simulink model "simulation"  (R2017b)
settings: Solver=FixedStepAuto  StartTime=0.0  StopTime=simTotalTime  FixedStep=0.05  MaxStep=0.1  MinStep=0.01  RelTol=1e-3
undefined symbols (not defined in the file): gridArea, gridDen, gridLength, hysteronMax, hysteronMin, initialRelays, inputFactor, inputMax, inputMin, offset, outputFactor, outputMax, outputMin, weightFunc, xyGrid
libraries: simulink x1
settings Model: Creator=Marco  LastModifiedBy=M. Vasquez Beltran

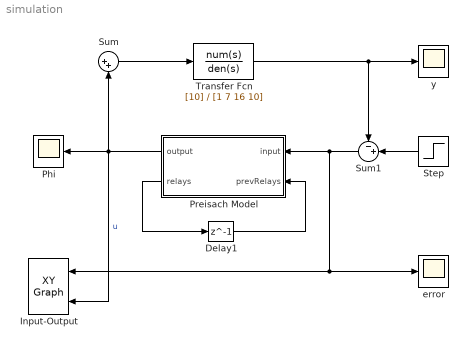
== system simulation ==
  Delay1 : Delay  DelayLength=1  InitialCondition=initialRelays
  Input-Output : simulink/Sinks/XY Graph  xmin=inputMin*inputFactor  xmax=inputMax*inputFactor  ymin=outputMin*outputFactor  ymax=outputMax*outputFactor  st=-1
  Phi : Scope
  Preisach Model : MATLAB Function  TreatAsAtomicUnit=on
  Step : Step  Time=100  After=-0.5  SampleTime=0
  Sum : Sum  Inputs=|++
  Sum1 : Sum  Inputs=-+|
  Transfer Fcn : TransferFcn  Numerator=[10]  Denominator=[1 7 16 10]
  error : Scope
  y : Scope
  wires:
  Preisach Model/2(relays) -> Delay1/1
  Delay1/1 -> Preisach Model/2(prevRelays)
  Preisach Model/1(output) -> Sum/2, Phi/1, Input-Output/2  "u"
  Sum/1 -> Transfer Fcn/1
  Transfer Fcn/1 -> Sum1/1, y/1
  Sum1/1 -> error/1, Input-Output/1, Preisach Model/1(input)
  Step/1 -> Sum1/2

== matlab function simulation/Preisach Model ==
  data: input input; prevRelays input; output output; weightFunc parameter; relays output; offset parameter; hysteronMin parameter; hysteronMax parameter; gridLength parameter; gridDen parameter; gridArea parameter; xyGrid parameter
function [output, relays] = fcn(input, prevRelays, ...
    weightFunc, offset, hysteronMin, hysteronMax, gridLength, gridDen, gridArea, xyGrid)

    output = offset;
    relays = prevRelays;
    for i=1:gridDen
        ii = gridDen-i+1; %index inversion for rows
        for j=1:i
            if( input >= xyGrid(i) && relays(ii,j) ~= hysteronMax )
                relays(ii,j) = hysteronMax;
            elseif( input <= xyGrid(j) && relays(ii,j) ~= hysteronMin )
                relays(ii,j) = hysteronMin;
            end
            output = output + relays(ii,j)*weightFunc(ii,j)*gridArea;
        end
    end
end
